simulink model "Copy_of_EMB_LRM_LaneRoleManager"  (R2025a)
settings: Solver=FixedStepDiscrete  StartTime=0.0  StopTime=inf  FixedStep=0.01  RelTol=1e-3
(part 1 of 2)
settings Model: Creator=wangtianqi  LastModifiedBy=wangtianqi

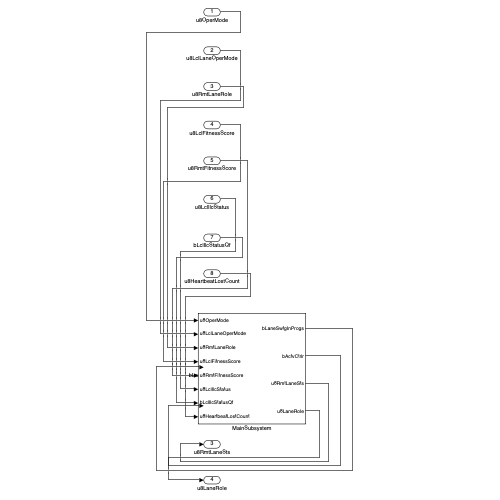
[thumbnail: Simulink's stored preview of the top-level diagram]
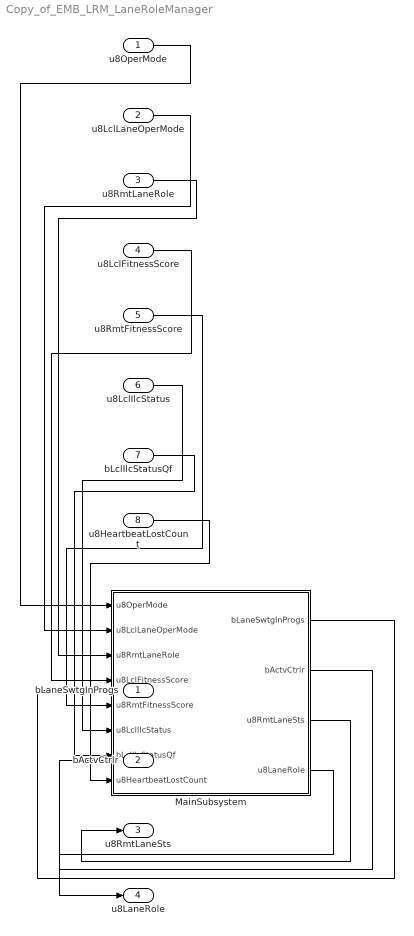
== system Copy_of_EMB_LRM_LaneRoleManager ==
  u8OperMode : Inport  Description=系统运行模式；类型 uint8；单位 -；范围 0..5 (0=OPMODE_INIT,1=OPMODE_NORMAL_OPERATION,2=OPMODE_LIMP_HOME,3=OPMODE_LIMP_ASIDE,4=OPMODE_CRAWL,5=OPMODE_SHUTTING_DOWN)  OutDataTypeStr=uint8
  u8LclLaneOperMode : Inport  Description=本控制链路运行模式；类型 uint8；单位 -；范围 0..5 (编码同系统运行模式)  Port=2  OutDataTypeStr=uint8
  u8RmtLaneRole : Inport  Description=远控制链路当前角色；类型 uint8；单位 -；范围 0..6 (0=UNKNOWN,1=INIT,2=MASTER,3=FALLBACK,4=SUPPORT,5=DISABLED,6=SHUTTING_DOWN)  Port=3  OutDataTypeStr=uint8
  u8LclFitnessScore : Inport  Description=本控制链路健康度得分；类型 uint8；单位 -；范围 0..255 (62=禁用,255=无效)  Port=4  OutDataTypeStr=uint8
  u8RmtFitnessScore : Inport  Description=远控制链路健康度得分；类型 uint8；单位 -；范围 0..255 (62=禁用,255=无效)  Port=5  OutDataTypeStr=uint8
  u8LclIlcStatus : Inport  Description=本控制链路 ILC 状态；类型 uint8；单位 -；范围 0..2 (0=Failed,1=Normal,2=Initialized)  Port=6  OutDataTypeStr=uint8
  bLclIlcStatusQf : Inport  Description=本控制链路 ILC 状态信号质量；类型 boolean；单位 -；范围 0..1 (1=QF_Not_Full 质量异常,0=QF_Full 质量正常)  Port=7  OutDataTypeStr=boolean
  u8HeartbeatLostCount : Inport  Description=心跳丢失计数；类型 uint8；单位 -；范围 0..255 (连续递增序列 0..255,0,1.. 表示正常)  Port=8  OutDataTypeStr=uint8
  MainSubsystem : Subsystem  Description=LRM 主包装子系统：信号采集 -> 链路状态管理(MLS) -> 角色仲裁(MLR) -> 切换防抖(LSP) -> 输出仲裁，实现 EMB 控制链路主从角色管理与切换标志输出
  bLaneSwtgInProgs : Outport  Description=控制链路切换进行中标志；类型 boolean；单位 -；范围 0..1 (0=Not Progress,1=Progress)
  bActvCtrlr : Outport  Description=活动控制器实例标志（本链路角色为 MASTER 时置 1）；类型 boolean；单位 -；范围 0..1 (0=Not Active,1=Active)  Port=2
  u8RmtLaneSts : Outport  Description=远控制链路状态（由远控角色与健康度映射派生）；类型 uint8；单位 -；范围 0..3 (0=INITIALISING,1=OPERATING,2=HB_LOST,3=FAILED)  Port=3
  u8LaneRole : Outport  Description=本控制链路角色状态；类型 uint8；单位 -；范围 0..6 (0=UNKNOWN,1=INIT,2=MASTER,3=FALLBACK,4=SUPPORT,5=DISABLED,6=SHUTTING_DOWN)  Port=4
  wires:
  u8OperMode/1 -> MainSubsystem/1(u8OperMode)
  u8LclLaneOperMode/1 -> MainSubsystem/2(u8LclLaneOperMode)
  u8RmtLaneRole/1 -> MainSubsystem/3(u8RmtLaneRole)
  u8LclFitnessScore/1 -> MainSubsystem/4(u8LclFitnessScore)
  u8RmtFitnessScore/1 -> MainSubsystem/5(u8RmtFitnessScore)
  u8LclIlcStatus/1 -> MainSubsystem/6(u8LclIlcStatus)
  bLclIlcStatusQf/1 -> MainSubsystem/7(bLclIlcStatusQf)
  u8HeartbeatLostCount/1 -> MainSubsystem/8(u8HeartbeatLostCount)
  MainSubsystem/1(bLaneSwtgInProgs) -> bLaneSwtgInProgs/1
  MainSubsystem/2(bActvCtrlr) -> bActvCtrlr/1
  MainSubsystem/3(u8RmtLaneSts) -> u8RmtLaneSts/1
  MainSubsystem/4(u8LaneRole) -> u8LaneRole/1

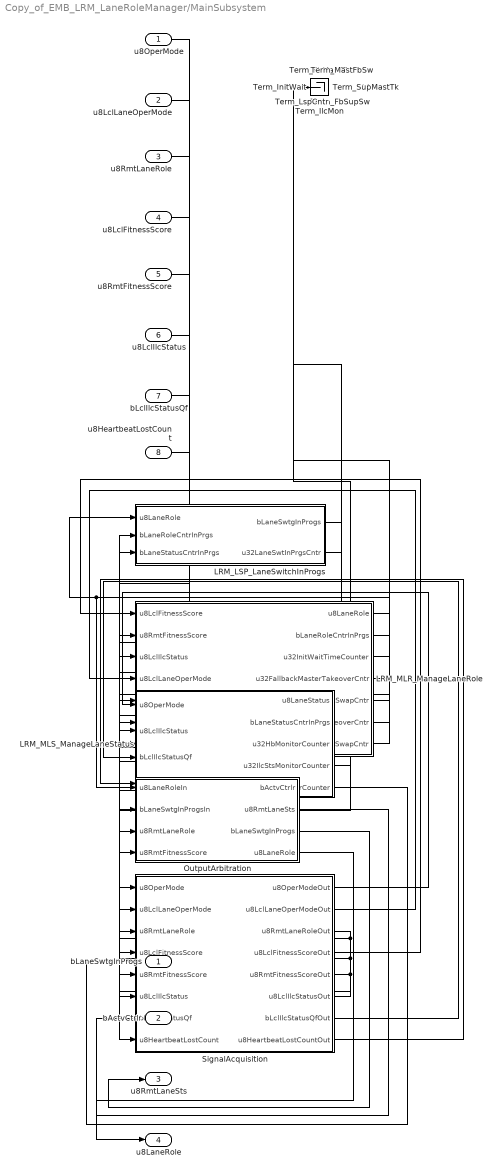
== system Copy_of_EMB_LRM_LaneRoleManager/MainSubsystem ==
  u8OperMode : Inport  Description=系统运行模式；类型 uint8；单位 -；范围 0..5  OutDataTypeStr=uint8
  u8LclLaneOperMode : Inport  Description=本控制链路运行模式；类型 uint8；单位 -；范围 0..5  Port=2  OutDataTypeStr=uint8
  u8RmtLaneRole : Inport  Description=远控制链路当前角色；类型 uint8；单位 -；范围 0..6  Port=3  OutDataTypeStr=uint8
  u8LclFitnessScore : Inport  Description=本控制链路健康度得分；类型 uint8；单位 -；范围 0..255 (62=禁用,255=无效)  Port=4  OutDataTypeStr=uint8
  u8RmtFitnessScore : Inport  Description=远控制链路健康度得分；类型 uint8；单位 -；范围 0..255 (62=禁用,255=无效)  Port=5  OutDataTypeStr=uint8
  u8LclIlcStatus : Inport  Description=本控制链路 ILC 状态；类型 uint8；单位 -；范围 0..2 (0=Failed,1=Normal,2=Initialized)  Port=6  OutDataTypeStr=uint8
  bLclIlcStatusQf : Inport  Description=本控制链路 ILC 状态信号质量；类型 boolean；单位 -；范围 0..1 (1=质量异常,0=质量正常)  Port=7  OutDataTypeStr=boolean
  u8HeartbeatLostCount : Inport  Description=心跳丢失计数；类型 uint8；单位 -；范围 0..255  Port=8  OutDataTypeStr=uint8
  LRM_LSP_LaneSwitchInProgs : Subsystem  Description=检测角色（LaneRole）变化并管理角色切换过渡过程（防抖），输出切换进行中标志与计数器；优先级 A>B>C：A=LaneRoleChanged 时 cntr=1,flag=1；B=cntr>0 时 cntr+1 并在超阈值后清零；C=IfAnyTimerNonZero 时 cntr=0,flag=1；由 Unit Delay / Sum / Switch 优先级链 / Relational Operator / Logical Operator 实现
  LRM_MLR_ManageLaneRole : Subsystem  Description=基于本/远控制链路健康度得分、ILC 状态、远控角色、LaneStatus 与运行模式仲裁本控制链路角色（INIT/DISABLED/SHUTTING_DOWN/SUPPORT/FALLBACK/MASTER）；内部含 MLR_STM（boolean-gated Stateflow，状态 Init/Disabled/ShuttingDown/OperationalRoles{Support,Fallback,Master}）与 Simulink 计数器（InitWaitTime/MasterFallbackSwap/FallbackMasterTakeover/FallbackSupportSwap/SupportMasterTakeover），条件全部在 Simulink 内计算为 boolean，图表仅输出 u8LaneRole
  LRM_MLS_ManageLaneStatus : Subsystem  Description=监控 LCL ILC STATUS_QF、OPER MODE 与 LCL ILC STATUS，结合心跳丢失判定输出控制链路健康状态 LaneStatus、状态切换标志与三个诊断计数器；内部含 MLS_HB_Failure（Unit Delay/Sum/Relational/Logic 组合）与 MLS_STM_StateMachine（boolean-gated Stateflow，状态 INIT.MonitoringOff/On、Operating、HbLost、Failed，优先级 Operating>Failed>HbLost；计数器与条件全部在 Simulink 内计算，图表仅接收 boolean 条件，输出 u8LaneStatus 与 bMonitoringActive）
  OutputArbitration : Subsystem  Description=输出仲裁与派生诊断：bActvCtrlr=(u8LaneRole==2)（Relational Operator）；u8RmtLaneSts 由 Switch 优先级链映射（DISABLED/SHUTTING_DOWN→FAILED、FITNESS==255→HB_LOST、UNKNOWN/INIT→INITIALISING、其余→OPERATING）；bLaneSwtgInProgs 与 u8LaneRole 直通
  SignalAcquisition : Subsystem  Description=信号调理与类型转换：全部顶层输入已采用内部一致表示（enum 用 uint8，质量标志用 boolean），无需类型转换，直通至下游；8 路输入与 8 路输出同名同类型一一对应，由同名 Inport/Outport 直连实现
  Term_FbMastTk : Terminator
      settings: Description=诊断计数器终止：u32FallbackMasterTakeoverCntr
  Term_FbSupSw : Terminator
      settings: Description=诊断计数器终止：u32FallbackSupportSwapCntr
  Term_HbMon : Terminator
      settings: Description=诊断计数器终止：u32HbMonitorCounter
  Term_IlcMon : Terminator
      settings: Description=诊断计数器终止：u32IlcStsMonitorCounter
  Term_InitWait : Terminator
      settings: Description=诊断计数器终止：u32InitWaitTimeCounter
  Term_LspCntr : Terminator
      settings: Description=诊断计数器终止：u32LaneSwtInPrgsCntr
  Term_MastFbSw : Terminator
      settings: Description=诊断计数器终止：u32MasterFallbackSwapCntr
  Term_SupMastTk : Terminator
      settings: Description=诊断计数器终止：u32SupportMasterTakeoverCntr
  bLaneSwtgInProgs : Outport  Description=控制链路切换进行中标志；类型 boolean；单位 -；范围 0..1
  bActvCtrlr : Outport  Description=活动控制器实例标志；类型 boolean；单位 -；范围 0..1  Port=2
  u8RmtLaneSts : Outport  Description=远控制链路状态；类型 uint8；单位 -；范围 0..3  Port=3
  u8LaneRole : Outport  Description=本控制链路角色状态；类型 uint8；单位 -；范围 0..6  Port=4
  wires:
  u8OperMode/1 -> SignalAcquisition/1(u8OperMode)
  u8LclLaneOperMode/1 -> SignalAcquisition/2(u8LclLaneOperMode)
  u8RmtLaneRole/1 -> SignalAcquisition/3(u8RmtLaneRole)
  u8LclFitnessScore/1 -> SignalAcquisition/4(u8LclFitnessScore)
  u8RmtFitnessScore/1 -> SignalAcquisition/5(u8RmtFitnessScore)
  u8LclIlcStatus/1 -> SignalAcquisition/6(u8LclIlcStatus)
  bLclIlcStatusQf/1 -> SignalAcquisition/7(bLclIlcStatusQf)
  u8HeartbeatLostCount/1 -> SignalAcquisition/8(u8HeartbeatLostCount)
  SignalAcquisition/1(u8OperModeOut) -> LRM_MLS_ManageLaneStatus/1(u8OperMode)
  SignalAcquisition/2(u8LclLaneOperModeOut) -> LRM_MLR_ManageLaneRole/4(u8LclLaneOperMode)
  SignalAcquisition/3(u8RmtLaneRoleOut) -> OutputArbitration/3(u8RmtLaneRole), LRM_MLR_ManageLaneRole/5(u8RmtLaneRole)
  SignalAcquisition/4(u8LclFitnessScoreOut) -> LRM_MLR_ManageLaneRole/1(u8LclFitnessScore)
  SignalAcquisition/5(u8RmtFitnessScoreOut) -> OutputArbitration/4(u8RmtFitnessScore), LRM_MLR_ManageLaneRole/2(u8RmtFitnessScore)
  SignalAcquisition/6(u8LclIlcStatusOut) -> LRM_MLR_ManageLaneRole/3(u8LclIlcStatus), LRM_MLS_ManageLaneStatus/2(u8LclIlcStatus)
  SignalAcquisition/7(bLclIlcStatusQfOut) -> LRM_MLS_ManageLaneStatus/3(bLclIlcStatusQf)
  SignalAcquisition/8(u8HeartbeatLostCountOut) -> LRM_MLS_ManageLaneStatus/4(u8HeartbeatLostCount)
  LRM_MLS_ManageLaneStatus/1(u8LaneStatus) -> LRM_MLR_ManageLaneRole/6(u8LaneStatus)
  LRM_MLS_ManageLaneStatus/2(bLaneStatusCntrInPrgs) -> LRM_LSP_LaneSwitchInProgs/3(bLaneStatusCntrInPrgs)
  LRM_MLS_ManageLaneStatus/3(u32HbMonitorCounter) -> Term_HbMon/1
  LRM_MLS_ManageLaneStatus/4(u32IlcStsMonitorCounter) -> Term_IlcMon/1
  LRM_MLS_ManageLaneStatus/5(u32FailureMonitorCounter) -> LRM_MLR_ManageLaneRole/7(u32FailureMonitorCounter)
  LRM_MLR_ManageLaneRole/1(u8LaneRole) -> LRM_LSP_LaneSwitchInProgs/1(u8LaneRole), OutputArbitration/1(u8LaneRoleIn)
  LRM_MLR_ManageLaneRole/2(bLaneRoleCntrInPrgs) -> LRM_LSP_LaneSwitchInProgs/2(bLaneRoleCntrInPrgs)
  LRM_MLR_ManageLaneRole/3(u32InitWaitTimeCounter) -> Term_InitWait/1
  LRM_MLR_ManageLaneRole/4(u32FallbackMasterTakeoverCntr) -> Term_FbMastTk/1
  LRM_MLR_ManageLaneRole/5(u32MasterFallbackSwapCntr) -> Term_MastFbSw/1
  LRM_MLR_ManageLaneRole/6(u32SupportMasterTakeoverCntr) -> Term_SupMastTk/1
  LRM_MLR_ManageLaneRole/7(u32FallbackSupportSwapCntr) -> Term_FbSupSw/1
  LRM_LSP_LaneSwitchInProgs/1(bLaneSwtgInProgs) -> OutputArbitration/2(bLaneSwtgInProgsIn)
  LRM_LSP_LaneSwitchInProgs/2(u32LaneSwtInPrgsCntr) -> Term_LspCntr/1
  OutputArbitration/1(bActvCtrlr) -> bLaneSwtgInProgs/1
  OutputArbitration/2(u8RmtLaneSts) -> bActvCtrlr/1
  OutputArbitration/3(bLaneSwtgInProgs) -> u8RmtLaneSts/1
  OutputArbitration/4(u8LaneRole) -> u8LaneRole/1

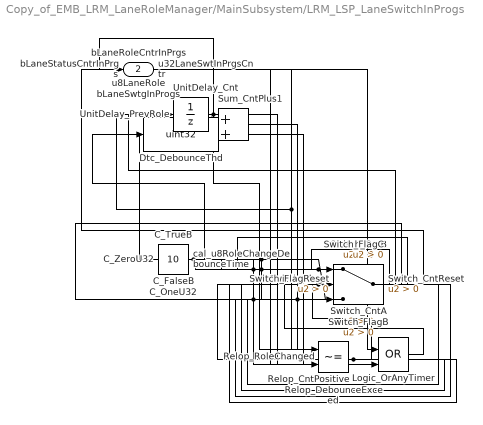
== system Copy_of_EMB_LRM_LaneRoleManager/MainSubsystem/LRM_LSP_LaneSwitchInProgs ==
  u8LaneRole : Inport  Description=当前周期角色决策值（来自 MLR）；类型 uint8；范围 0..6  OutDataTypeStr=uint8
  bLaneRoleCntrInPrgs : Inport  Description=角色切换计数器进行中标志（来自 MLR）；类型 boolean  Port=2  OutDataTypeStr=boolean
  bLaneStatusCntrInPrgs : Inport  Description=状态切换计数器进行中标志（来自 MLS）；类型 boolean  Port=3  OutDataTypeStr=boolean
  C_FalseB : Constant  Description=布尔假常量  Value=0  OutDataTypeStr=boolean
  C_OneU32 : Constant  Description=计数器步长 1；uint32  OutDataTypeStr=uint32
  C_TrueB : Constant  Description=布尔真常量  OutDataTypeStr=boolean
  C_ZeroU32 : Constant  Description=计数器清零常量；uint32  Value=0  OutDataTypeStr=uint32
  Dtc_DebounceThd : DataTypeConversion  Description=防抖阈值转 uint32  OutDataTypeStr=uint32  SaturateOnIntegerOverflow=off  RndMeth=Floor
  Logic_OrAnyTimer : Logic  Description=任一计时器进行中  Operator=OR  IconShape=distinctive  AllPortsSameDT=off  OutDataTypeStr=boolean
  Relop_CntPositive : RelationalOperator  Description=计数器 > 0（条件 B）  Operator=>  OutDataTypeStr=boolean  RndMeth=Simplest  InputSameDT=off
  Relop_DebounceExceed : RelationalOperator  Description=cnt+1 > 防抖阈值（清零条件）  Operator=>  OutDataTypeStr=boolean  RndMeth=Simplest  InputSameDT=off
  Relop_RoleChanged : RelationalOperator  Description=角色变化检测：当前角色 != 上一周期角色  Operator=~=  OutDataTypeStr=boolean  RndMeth=Simplest  InputSameDT=off
  Sum_CntPlus1 : Sum  Description=切换计数器 +1  Inputs=|++
  Switch_CntA : Switch  Description=A 优先级：角色变化置 1  Criteria=u2 > Threshold  SaturateOnIntegerOverflow=off  InputSameDT=off
  Switch_CntB : Switch  Description=B 分支门控：cnt>0 时按 B 处理，否则 0  Criteria=u2 > Threshold  SaturateOnIntegerOverflow=off  InputSameDT=off
  Switch_CntReset : Switch  Description=B 分支：超阈值清零，否则 +1  Criteria=u2 > Threshold  SaturateOnIntegerOverflow=off  InputSameDT=off
  Switch_FlagA : Switch  Description=标志 A 优先级：角色变化置 1  Criteria=u2 > Threshold  SaturateOnIntegerOverflow=off  InputSameDT=off
  Switch_FlagB : Switch  Description=标志 B 门控  Criteria=u2 > Threshold  SaturateOnIntegerOverflow=off  InputSameDT=off
  Switch_FlagC : Switch  Description=标志 C 分支：任一计时器进行中置 1  Criteria=u2 > Threshold  SaturateOnIntegerOverflow=off  InputSameDT=off
  Switch_FlagReset : Switch  Description=标志 B 分支：超阈值清零  Criteria=u2 > Threshold  SaturateOnIntegerOverflow=off  InputSameDT=off
  UnitDelay_Cnt : UnitDelay  Description=切换进行中计数器状态；uint32  SampleTime=-1  HasFrameUpgradeWarning=on
  UnitDelay_PrevRole : UnitDelay  Description=上一周期角色；uint8  SampleTime=-1  HasFrameUpgradeWarning=on
  cal_u8RoleChangeDebounceTime : Constant  Description=cal_u8RoleChangeDebounceTime；角色切换防抖时间阈值（周期数）；uint8；1..255；默认 10  Value=10  OutDataTypeStr=uint8
  bLaneSwtgInProgs : Outport  Description=控制链路切换进行中标志；类型 boolean；范围 0..1
  u32LaneSwtInPrgsCntr : Outport  Description=控制链路切换进行中计数器；类型 uint32  Port=2
  wires:
  u8LaneRole/1 -> UnitDelay_PrevRole/1, Relop_RoleChanged/1
  UnitDelay_PrevRole/1 -> Relop_RoleChanged/2
  bLaneRoleCntrInPrgs/1 -> Logic_OrAnyTimer/1
  bLaneStatusCntrInPrgs/1 -> Logic_OrAnyTimer/2
  UnitDelay_Cnt/1 -> Relop_CntPositive/1, Sum_CntPlus1/1, u32LaneSwtInPrgsCntr/1
  C_OneU32/1 -> Switch_CntA/1, Sum_CntPlus1/2
  C_ZeroU32/1 -> Switch_CntB/3, Relop_CntPositive/2, Switch_CntReset/1
  cal_u8RoleChangeDebounceTime/1 -> Dtc_DebounceThd/1
  Dtc_DebounceThd/1 -> Relop_DebounceExceed/2
  Sum_CntPlus1/1 -> Switch_CntReset/3, Relop_DebounceExceed/1
  Relop_DebounceExceed/1 -> Switch_FlagReset/2, Switch_CntReset/2
  Switch_CntReset/1 -> Switch_CntB/1
  Relop_CntPositive/1 -> Switch_FlagB/2, Switch_CntB/2
  Relop_RoleChanged/1 -> Switch_FlagA/2, Switch_CntA/2
  Switch_CntB/1 -> Switch_CntA/3
  Switch_CntA/1 -> UnitDelay_Cnt/1
  C_FalseB/1 -> Switch_FlagC/3, Switch_FlagReset/1
  C_TrueB/1 -> Switch_FlagA/1, Switch_FlagC/1, Switch_FlagReset/3
  Switch_FlagReset/1 -> Switch_FlagB/1
  Switch_FlagC/1 -> Switch_FlagB/3
  Logic_OrAnyTimer/1 -> Switch_FlagC/2
  Switch_FlagB/1 -> Switch_FlagA/3
  Switch_FlagA/1 -> bLaneSwtgInProgs/1

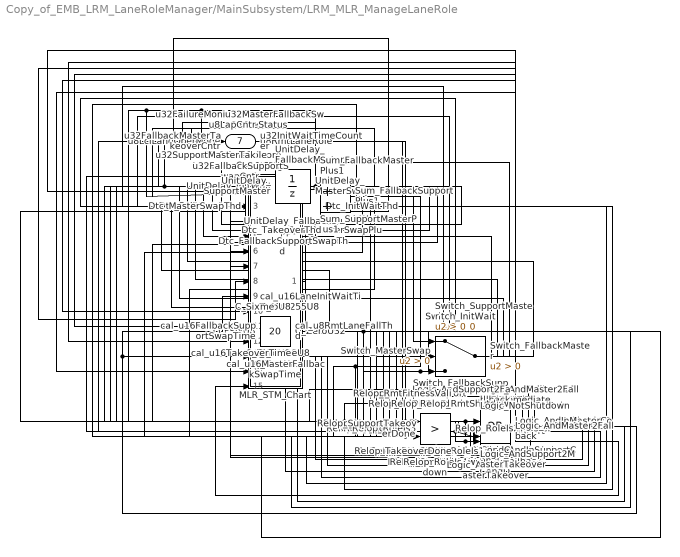
== system Copy_of_EMB_LRM_LaneRoleManager/MainSubsystem/LRM_MLR_ManageLaneRole ==
  u8LclFitnessScore : Inport  Description=本控制链路健康度得分；类型 uint8；范围 0..255 (62=禁用,255=无效)  OutDataTypeStr=uint8
  u8RmtFitnessScore : Inport  Description=远控制链路健康度得分；类型 uint8；范围 0..255 (62=禁用,255=无效)  Port=2  OutDataTypeStr=uint8
  u8LclIlcStatus : Inport  Description=本控制链路 ILC 状态；类型 uint8；范围 0..2 (0=Failed,1=Normal,2=Initialized)  Port=3  OutDataTypeStr=uint8
  u8LclLaneOperMode : Inport  Description=本控制链路运行模式；类型 uint8；范围 0..5  Port=4  OutDataTypeStr=uint8
  u8RmtLaneRole : Inport  Description=远控制链路当前角色；类型 uint8；范围 0..6  Port=5  OutDataTypeStr=uint8
  u8LaneStatus : Inport  Description=控制链路健康状态（来自 MLS）；类型 uint8；范围 0..3  Port=6  OutDataTypeStr=uint8
  u32FailureMonitorCounter : Inport  Description=故障监控计数器（来自 MLS）；类型 uint32  Port=7  OutDataTypeStr=uint32
  C_FiveU8 : Constant  Description=常量 5（LN_ROLE_DISABLED）；uint8  Value=5  OutDataTypeStr=uint8
  C_FourU8 : Constant  Description=常量 4（LN_ROLE_SUPPORT）；uint8  Value=4  OutDataTypeStr=uint8
  C_Max255U8 : Constant  Description=健康度无效值 255；uint8  Value=255  OutDataTypeStr=uint8
  C_OneU32 : Constant  Description=计数器步长 1；uint32  OutDataTypeStr=uint32
  C_OneU8 : Constant  Description=常量 1（LN_ROLE_INIT）；uint8  OutDataTypeStr=uint8
  C_SixTwoU8 : Constant  Description=健康度禁用值 62；uint8  Value=62  OutDataTypeStr=uint8
  C_SixU8 : Constant  Description=常量 6（LN_ROLE_SHUTTING_DOWN）；uint8  Value=6  OutDataTypeStr=uint8
  C_ThreeU8 : Constant  Description=常量 3（LN_ROLE_FALLBACK）；uint8  Value=3  OutDataTypeStr=uint8
  C_TwoU8 : Constant  Description=常量 2（LN_ROLE_MASTER）；uint8  Value=2  OutDataTypeStr=uint8
  C_ZeroU32 : Constant  Description=计数器清零常量；uint32  Value=0  OutDataTypeStr=uint32
  C_ZeroU8 : Constant  Description=零常量；uint8  Value=0  OutDataTypeStr=uint8
  Dtc_FailWatchThd : DataTypeConversion  Description=故障监控阈值转 uint32  OutDataTypeStr=uint32  SaturateOnIntegerOverflow=off  RndMeth=Floor
  Dtc_FallbackSupportSwapThd : DataTypeConversion  Description=FallbackSupportSwap 阈值转 uint32  OutDataTypeStr=uint32  SaturateOnIntegerOverflow=off  RndMeth=Floor
  Dtc_InitWaitThd : DataTypeConversion  Description=InitWait 阈值转 uint32  OutDataTypeStr=uint32  SaturateOnIntegerOverflow=off  RndMeth=Floor
  Dtc_MasterSwapThd : DataTypeConversion  Description=MasterSwap 阈值转 uint32  OutDataTypeStr=uint32  SaturateOnIntegerOverflow=off  RndMeth=Floor
  Dtc_TakeoverThd : DataTypeConversion  Description=接管阈值转 uint32  OutDataTypeStr=uint32  SaturateOnIntegerOverflow=off  RndMeth=Floor
  Logic_AndArbLcl : Logic  Description=仲裁条件（本地更优）：等待完成 且 本地>远程  IconShape=distinctive  AllPortsSameDT=off  OutDataTypeStr=boolean
  Logic_AndCondA : Logic  Description=条件A：ILC 故障 且 远程有效 且 本地<远程（Master->Support 直接降级）  Inputs=3  IconShape=distinctive  AllPortsSameDT=off  OutDataTypeStr=boolean
  Logic_AndCondD : Logic  Description=条件D：本地>远程 且 远程有效（接管条件，假设）  IconShape=distinctive  AllPortsSameDT=off  OutDataTypeStr=boolean
  Logic_AndFallback2MasterTakeover : Logic  Description=Fallback->Master（接管）：条件D 且 计数超阈值 且 远程非MASTER  Inputs=3  IconShape=distinctive  AllPortsSameDT=off  OutDataTypeStr=boolean
  Logic_AndFallback2Support : Logic  Description=Fallback->Support：条件E 且 计数超阈值  IconShape=distinctive  AllPortsSameDT=off  OutDataTypeStr=boolean
  Logic_AndFallback2SupportUnknown : Logic  Description=Fallback->Support：远程UNKNOWN 且 故障监控超窗  IconShape=distinctive  AllPortsSameDT=off  OutDataTypeStr=boolean
  Logic_AndInFallbackCondD : Logic  Description=Fallback 内条件D持续  IconShape=distinctive  AllPortsSameDT=off  OutDataTypeStr=boolean
  Logic_AndInFallbackCondE : Logic  Description=Fallback 内条件E持续  IconShape=distinctive  AllPortsSameDT=off  OutDataTypeStr=boolean
  Logic_AndInMasterCondB : Logic  Description=Master 内条件B持续  IconShape=distinctive  AllPortsSameDT=off  OutDataTypeStr=boolean
  Logic_AndInSupportCondG : Logic  Description=Support 内条件G持续  IconShape=distinctive  AllPortsSameDT=off  OutDataTypeStr=boolean
  Logic_AndMaster2Fallback : Logic  Description=Master->Fallback：条件B持续 且 远程FALLBACK 且 计数超阈值  Inputs=3  IconShape=distinctive  AllPortsSameDT=off  OutDataTypeStr=boolean
  Logic_AndMaster2FallbackImmediate : Logic  Description=Master->Fallback（立即）：条件B 且 远程MASTER  IconShape=distinctive  AllPortsSameDT=off  OutDataTypeStr=boolean
  Logic_AndSupport2Fallback : Logic  Description=Support->Fallback（恢复）：ILC 非故障 且 远程MASTER  IconShape=distinctive  AllPortsSameDT=off  OutDataTypeStr=boolean
  Logic_AndSupport2MasterTakeover : Logic  Description=Support->Master（接管）：条件G 且 计数超阈值 且 远程非MASTER  Inputs=3  IconShape=distinctive  AllPortsSameDT=off  OutDataTypeStr=boolean
  Logic_NotIlcFailed : Logic  Description=ILC 非 Failed  Operator=NOT  Inputs=1  IconShape=distinctive  AllPortsSameDT=off  OutDataTypeStr=boolean
  Logic_NotShutdown : Logic  Description=非关闭模式  Operator=NOT  Inputs=1  IconShape=distinctive  AllPortsSameDT=off  OutDataTypeStr=boolean
  Logic_OrCondC : Logic  Description=条件C：LaneStatus==FAILED 或 远程禁用/关闭  Operator=OR  IconShape=distinctive  AllPortsSameDT=off  OutDataTypeStr=boolean
  Logic_OrRmtDisShut : Logic  Description=远程禁用或关闭  Operator=OR  IconShape=distinctive  AllPortsSameDT=off  OutDataTypeStr=boolean
  MLR_STM_Chart : Stateflow chart  Description=MLR_STM 布尔门控 Stateflow：输入全为 boolean 条件（15 路），输出 u8LaneRole；状态 Init/Disabled/ShuttingDown/OperationalRoles{Support,FallBack,Master}  TreatAsAtomicUnit=on
  Relop_FailWatchDone : RelationalOperator  Description=FailureMonitorCounter > 窗口阈值  Operator=>  OutDataTypeStr=boolean  RndMeth=Simplest  InputSameDT=off
  Relop_FallbackSwapDone : RelationalOperator  Description=FallbackSupportSwapCntr > 阈值  Operator=>  OutDataTypeStr=boolean  RndMeth=Simplest  InputSameDT=off
  Relop_IlcFailed : RelationalOperator  Description=ILC 状态==Failed  Operator===  OutDataTypeStr=boolean  RndMeth=Simplest  InputSameDT=off
  Relop_InitWaitDone : RelationalOperator  Description=InitWaitTime >= 阈值  Operator=<=  OutDataTypeStr=boolean  RndMeth=Simplest  InputSameDT=off
  Relop_LaneOperShutdown : RelationalOperator  Description=本链路运行模式==SHUTTING_DOWN  Operator===  OutDataTypeStr=boolean  RndMeth=Simplest  InputSameDT=off
  Relop_LaneStsFailed : RelationalOperator  Description=LaneStatus==FAILED  Operator===  OutDataTypeStr=boolean  RndMeth=Simplest  InputSameDT=off
  Relop_LclDisabled : RelationalOperator  Description=本链路健康度==62（禁用）  Operator===  OutDataTypeStr=boolean  RndMeth=Simplest  InputSameDT=off
  Relop_LclGtRmt : RelationalOperator  Description=本链路健康度 > 远程  Operator=>  OutDataTypeStr=boolean  RndMeth=Simplest  InputSameDT=off
  Relop_LclLtRmt : RelationalOperator  Description=本链路健康度 < 远程  Operator=<  OutDataTypeStr=boolean  RndMeth=Simplest  InputSameDT=off
  Relop_MasterSwapDone : RelationalOperator  Description=MasterSwapCntr > 阈值  Operator=>  OutDataTypeStr=boolean  RndMeth=Simplest  InputSameDT=off
  Relop_RmtDisabled : RelationalOperator  Description=远程角色==DISABLED  Operator===  OutDataTypeStr=boolean  RndMeth=Simplest  InputSameDT=off
  Relop_RmtFallback : RelationalOperator  Description=远程角色==FALLBACK  Operator===  OutDataTypeStr=boolean  RndMeth=Simplest  InputSameDT=off
  Relop_RmtFitnessValid : RelationalOperator  Description=远程健康度非无效(255)  Operator=~=  OutDataTypeStr=boolean  RndMeth=Simplest  InputSameDT=off
  Relop_RmtMaster : RelationalOperator  Description=远程角色==MASTER  Operator===  OutDataTypeStr=boolean  RndMeth=Simplest  InputSameDT=off
  Relop_RmtNotMaster : RelationalOperator  Description=远程角色非 MASTER  Operator=~=  OutDataTypeStr=boolean  RndMeth=Simplest  InputSameDT=off
  Relop_RmtShutdown : RelationalOperator  Description=远程角色==SHUTTING_DOWN  Operator===  OutDataTypeStr=boolean  RndMeth=Simplest  InputSameDT=off
  Relop_RmtUnknown : RelationalOperator  Description=远程角色==UNKNOWN  Operator===  OutDataTypeStr=boolean  RndMeth=Simplest  InputSameDT=off
  Relop_RoleIs1 : RelationalOperator  Description=当前角色==INIT  Operator===  OutDataTypeStr=boolean  RndMeth=Simplest  InputSameDT=off
  Relop_RoleIs2 : RelationalOperator  Description=当前角色==MASTER  Operator===  OutDataTypeStr=boolean  RndMeth=Simplest  InputSameDT=off
  Relop_RoleIs3 : RelationalOperator  Description=当前角色==FALLBACK  Operator===  OutDataTypeStr=boolean  RndMeth=Simplest  InputSameDT=off
  Relop_RoleIs4 : RelationalOperator  Description=当前角色==SUPPORT  Operator===  OutDataTypeStr=boolean  RndMeth=Simplest  InputSameDT=off
  Relop_SupportTakeoverDone : RelationalOperator  Description=SupportMasterTakeoverCntr > 阈值  Operator=>  OutDataTypeStr=boolean  RndMeth=Simplest  InputSameDT=off
  Relop_TakeoverDone : RelationalOperator  Description=FallbackMasterTakeoverCntr > 阈值  Operator=>  OutDataTypeStr=boolean  RndMeth=Simplest  InputSameDT=off
  Sum_FallbackMasterPlus1 : Sum  Description=FallbackMaster 计数器 +1  Inputs=|++
  Sum_FallbackSupportPlus1 : Sum  Description=FallbackSupport 计数器 +1  Inputs=|++
  Sum_InitWaitPlus1 : Sum  Description=InitWait 计数器 +1  Inputs=|++
  Sum_MasterSwapPlus1 : Sum  Description=MasterSwap 计数器 +1  Inputs=|++
  Sum_SupportMasterPlus1 : Sum  Description=SupportMaster 计数器 +1  Inputs=|++
  Switch_FallbackMaster : Switch  Description=Fallback 内条件D持续时计数，否则清零  Criteria=u2 > Threshold  SaturateOnIntegerOverflow=off  InputSameDT=off
  Switch_FallbackSupport : Switch  Description=Fallback 内条件E持续时计数，否则清零  Criteria=u2 > Threshold  SaturateOnIntegerOverflow=off  InputSameDT=off
  Switch_InitWait : Switch  Description=Init 状态内计数，否则清零  Criteria=u2 > Threshold  SaturateOnIntegerOverflow=off  InputSameDT=off
  Switch_MasterSwap : Switch  Description=Master 内条件B持续时计数，否则清零  Criteria=u2 > Threshold  SaturateOnIntegerOverflow=off  InputSameDT=off
  Switch_SupportMaster : Switch  Description=Support 内条件G持续时计数，否则清零  Criteria=u2 > Threshold  SaturateOnIntegerOverflow=off  InputSameDT=off
  UnitDelay_FallbackMaster : UnitDelay  Description=Fallback->Master 接管计数器；uint32  SampleTime=-1  HasFrameUpgradeWarning=on
  UnitDelay_FallbackSupport : UnitDelay  Description=Fallback->Support 切换计数器；uint32  SampleTime=-1  HasFrameUpgradeWarning=on
  UnitDelay_InitWait : UnitDelay  Description=初始化等待计数器状态；uint32  SampleTime=-1  HasFrameUpgradeWarning=on
  UnitDelay_MasterSwap : UnitDelay  Description=Master->Fallback 切换计数器；uint32  SampleTime=-1  HasFrameUpgradeWarning=on
  UnitDelay_SupportMaster : UnitDelay  Description=Support->Master 接管计数器；uint32  SampleTime=-1  HasFrameUpgradeWarning=on
  cal_u16FallbackSupportSwapTime : Constant  Description=cal_u16FallbackSupportSwapTime；Fallback->Support 切换阈值；uint16；1..65535；默认 20（假设值）  Value=20  OutDataTypeStr=uint16
  cal_u16LaneInitWaitTime : Constant  Description=cal_u16LaneInitWaitTime；初始化等待时间阈值（周期数）；uint16；1..65535；默认 100（假设值，文档未给初值）  Value=100  OutDataTypeStr=uint16
  cal_u16MasterFallbackSwapTime : Constant  Description=cal_u16MasterFallbackSwapTime；Master->Fallback 切换阈值；uint16；1..65535；默认 20  Value=20  OutDataTypeStr=uint16
  cal_u16TakeoverTime : Constant  Description=cal_u16TakeoverTime；接管计数阈值（周期数）；uint16；1..65535；默认 50（假设值）  Value=50  OutDataTypeStr=uint16
  cal_u8RmtLaneFallThd : Constant  Description=cal_u8RmtLaneFallThd；故障监控窗口阈值（周期数）；uint8；1..255；默认 20  Value=20  OutDataTypeStr=uint8
  u8LaneRole : Outport  Description=本控制链路角色决策结果；类型 uint8；范围 0..6
  bLaneRoleCntrInPrgs : Outport  Description=角色切换计数器进行中标志；类型 boolean  Port=2
  u32InitWaitTimeCounter : Outport  Description=初始化等待计数器；类型 uint32  Port=3
  u32FallbackMasterTakeoverCntr : Outport  Description=Fallback->Master 接管计数器；类型 uint32  Port=4
  u32MasterFallbackSwapCntr : Outport  Description=Master->Fallback 切换计数器；类型 uint32  Port=5
  u32SupportMasterTakeoverCntr : Outport  Description=Support->Master 接管计数器；类型 uint32  Port=6
  u32FallbackSupportSwapCntr : Outport  Description=Fallback->Support 切换计数器；类型 uint32  Port=7
  wires:
  u8LclFitnessScore/1 -> Relop_LclLtRmt/1, Relop_LclGtRmt/1, Relop_LclDisabled/1
  u8RmtFitnessScore/1 -> Relop_LclLtRmt/2, Relop_LclGtRmt/2, Relop_RmtFitnessValid/1
  u8LclIlcStatus/1 -> Relop_IlcFailed/1
  u8LclLaneOperMode/1 -> Relop_LaneOperShutdown/1
  u8RmtLaneRole/1 -> Relop_RmtUnknown/1, Relop_RmtShutdown/1, Relop_RmtDisabled/1, Relop_RmtNotMaster/1, Relop_RmtFallback/1, Relop_RmtMaster/1
  u8LaneStatus/1 -> Relop_LaneStsFailed/1
  u32FailureMonitorCounter/1 -> Relop_FailWatchDone/1
  C_SixTwoU8/1 -> Relop_LclDisabled/2
  C_Max255U8/1 -> Relop_RmtFitnessValid/2
  C_ZeroU8/1 -> Relop_RmtUnknown/2, Relop_IlcFailed/2
  C_FiveU8/1 -> Relop_RmtDisabled/2, Relop_LaneOperShutdown/2
  C_SixU8/1 -> Relop_RmtShutdown/2
  C_TwoU8/1 -> Relop_RoleIs2/2, Relop_RmtNotMaster/2, Relop_RmtMaster/2
  C_ThreeU8/1 -> Relop_RoleIs3/2, Relop_LaneStsFailed/2, Relop_RmtFallback/2
  Relop_LaneOperShutdown/1 -> Logic_NotShutdown/1, MLR_STM_Chart/1(bShutdown)
  Relop_RmtDisabled/1 -> Logic_OrRmtDisShut/1
  Relop_RmtShutdown/1 -> Logic_OrRmtDisShut/2
  Relop_LaneStsFailed/1 -> Logic_OrCondC/1
  Logic_OrRmtDisShut/1 -> Logic_OrCondC/2
  Relop_IlcFailed/1 -> Logic_AndInFallbackCondE/2, Logic_AndFallback2Support/1, Logic_AndCondA/1, Logic_NotIlcFailed/1
  Relop_RmtFitnessValid/1 -> Logic_AndCondD/2, Logic_AndCondA/2
  Relop_LclLtRmt/1 -> Logic_AndInMasterCondB/2, Logic_AndMaster2FallbackImmediate/1, Logic_AndMaster2Fallback/1, Logic_AndCondA/3
  Relop_LclGtRmt/1 -> Logic_AndArbLcl/2, Logic_AndCondD/1
  Relop_RmtFallback/1 -> Logic_AndMaster2Fallback/2
  Relop_MasterSwapDone/1 -> Logic_AndMaster2Fallback/3
  Relop_RmtMaster/1 -> Logic_AndSupport2Fallback/2, Logic_AndMaster2FallbackImmediate/2, MLR_STM_Chart/5(bArbRmtMaster)
  Logic_AndCondD/1 -> Logic_AndInSupportCondG/2, Logic_AndInFallbackCondD/2, Logic_AndSupport2MasterTakeover/1, Logic_AndFallback2MasterTakeover/1
  Relop_TakeoverDone/1 -> Logic_AndFallback2MasterTakeover/2
  Relop_RmtNotMaster/1 -> Logic_AndSupport2MasterTakeover/3, Logic_AndFallback2MasterTakeover/3
  Relop_FallbackSwapDone/1 -> Logic_AndFallback2Support/2
  Relop_RmtUnknown/1 -> Logic_AndFallback2SupportUnknown/1
  Relop_FailWatchDone/1 -> Logic_AndFallback2SupportUnknown/2
  Relop_SupportTakeoverDone/1 -> Logic_AndSupport2MasterTakeover/2
  Logic_NotIlcFailed/1 -> Logic_AndSupport2Fallback/1
  UnitDelay_InitWait/1 -> Relop_InitWaitDone/1, Sum_InitWaitPlus1/1, u32InitWaitTimeCounter/1
  C_OneU32/1 -> Sum_SupportMasterPlus1/2, Sum_FallbackSupportPlus1/2, Sum_FallbackMasterPlus1/2, Sum_MasterSwapPlus1/2, Sum_InitWaitPlus1/2
  Sum_InitWaitPlus1/1 -> Switch_InitWait/1
  Relop_RoleIs1/1 -> bLaneRoleCntrInPrgs/1, Switch_InitWait/2
  C_ZeroU32/1 -> Switch_SupportMaster/3, Switch_FallbackSupport/3, Switch_FallbackMaster/3, Switch_MasterSwap/3, Switch_InitWait/3
  Switch_InitWait/1 -> UnitDelay_InitWait/1
  Relop_RoleIs2/1 -> Logic_AndInMasterCondB/1
  UnitDelay_MasterSwap/1 -> Relop_MasterSwapDone/1, u32MasterFallbackSwapCntr/1, Sum_MasterSwapPlus1/1
  Sum_MasterSwapPlus1/1 -> Switch_MasterSwap/1
  Logic_AndInMasterCondB/1 -> Switch_MasterSwap/2
  Switch_MasterSwap/1 -> UnitDelay_MasterSwap/1
  Relop_RoleIs3/1 -> Logic_AndInFallbackCondE/1, Logic_AndInFallbackCondD/1
  UnitDelay_FallbackMaster/1 -> Relop_TakeoverDone/1, u32FallbackMasterTakeoverCntr/1, Sum_FallbackMasterPlus1/1
  Sum_FallbackMasterPlus1/1 -> Switch_FallbackMaster/1
  Logic_AndInFallbackCondD/1 -> Switch_FallbackMaster/2
  Switch_FallbackMaster/1 -> UnitDelay_FallbackMaster/1
  UnitDelay_FallbackSupport/1 -> Relop_FallbackSwapDone/1, u32FallbackSupportSwapCntr/1, Sum_FallbackSupportPlus1/1
  Sum_FallbackSupportPlus1/1 -> Switch_FallbackSupport/1
  Logic_AndInFallbackCondE/1 -> Switch_FallbackSupport/2
  Switch_FallbackSupport/1 -> UnitDelay_FallbackSupport/1
  Relop_RoleIs4/1 -> Logic_AndInSupportCondG/1
  UnitDelay_SupportMaster/1 -> Relop_SupportTakeoverDone/1, u32SupportMasterTakeoverCntr/1, Sum_SupportMasterPlus1/1
  Sum_SupportMasterPlus1/1 -> Switch_SupportMaster/1
  Logic_AndInSupportCondG/1 -> Switch_SupportMaster/2
  Switch_SupportMaster/1 -> UnitDelay_SupportMaster/1
  cal_u16LaneInitWaitTime/1 -> Dtc_InitWaitThd/1
  Dtc_InitWaitThd/1 -> Relop_InitWaitDone/2
  Relop_InitWaitDone/1 -> Logic_AndArbLcl/1
  cal_u16MasterFallbackSwapTime/1 -> Dtc_MasterSwapThd/1
  Dtc_MasterSwapThd/1 -> Relop_MasterSwapDone/2
  cal_u16TakeoverTime/1 -> Dtc_TakeoverThd/1
  Dtc_TakeoverThd/1 -> Relop_SupportTakeoverDone/2, Relop_TakeoverDone/2
  cal_u16FallbackSupportSwapTime/1 -> Dtc_FallbackSupportSwapThd/1
  Dtc_FallbackSupportSwapThd/1 -> Relop_FallbackSwapDone/2
  cal_u8RmtLaneFallThd/1 -> Dtc_FailWatchThd/1
  Dtc_FailWatchThd/1 -> Relop_FailWatchDone/2
  Logic_NotShutdown/1 -> MLR_STM_Chart/2(bNotShutdown)
  Relop_LclDisabled/1 -> MLR_STM_Chart/3(bLclDisabled)
  Logic_AndArbLcl/1 -> MLR_STM_Chart/4(bArbLclGtRmt)
  Logic_AndCondA/1 -> MLR_STM_Chart/6(bMaster2Support)
  Logic_AndMaster2Fallback/1 -> MLR_STM_Chart/7(bMaster2Fallback)
  Logic_AndMaster2FallbackImmediate/1 -> MLR_STM_Chart/8(bMaster2FallbackImmediate)
  Logic_OrCondC/1 -> MLR_STM_Chart/9(bFallback2Master), MLR_STM_Chart/13(bSupport2Master)
  Logic_AndFallback2MasterTakeover/1 -> MLR_STM_Chart/10(bFallback2MasterTakeover)
  Logic_AndFallback2Support/1 -> MLR_STM_Chart/11(bFallback2Support)
  Logic_AndFallback2SupportUnknown/1 -> MLR_STM_Chart/12(bFallback2SupportUnknown)
  Logic_AndSupport2MasterTakeover/1 -> MLR_STM_Chart/14(bSupport2MasterTakeover)
  Logic_AndSupport2Fallback/1 -> MLR_STM_Chart/15(bSupport2Fallback)
  MLR_STM_Chart/1(u8LaneRole) -> Relop_RoleIs4/1, Relop_RoleIs3/1, Relop_RoleIs2/1, Relop_RoleIs1/1, u8LaneRole/1
  C_OneU8/1 -> Relop_RoleIs1/2
  C_FourU8/1 -> Relop_RoleIs4/2

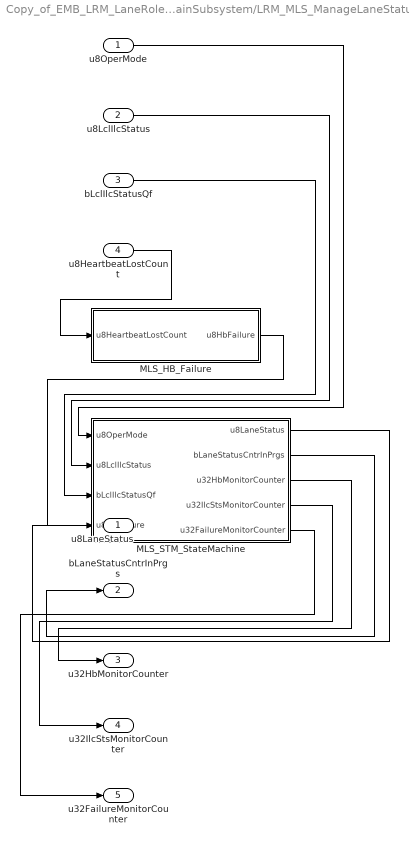
== system Copy_of_EMB_LRM_LaneRoleManager/MainSubsystem/LRM_MLS_ManageLaneStatus ==
  u8OperMode : Inport  Description=系统运行模式；类型 uint8；范围 0..5  OutDataTypeStr=uint8
  u8LclIlcStatus : Inport  Description=本控制链路 ILC 状态；类型 uint8；范围 0..2 (0=Failed,1=Normal,2=Initialized)  Port=2  OutDataTypeStr=uint8
  bLclIlcStatusQf : Inport  Description=本控制链路 ILC 状态信号质量；类型 boolean；范围 0..1 (1=异常,0=正常)  Port=3  OutDataTypeStr=boolean
  u8HeartbeatLostCount : Inport  Description=心跳丢失计数；类型 uint8；范围 0..255  Port=4  OutDataTypeStr=uint8
  MLS_HB_Failure : Subsystem  Description=MLS_HB_Failure 心跳丢失判定：HEARTBEAT LOST COUNT 连续递增(0..255,0,1..) 时 u8HbFailure=0，否则=1；由 Unit Delay 保存上一周期值，Sum/Relational Operator/Logical Operator 组合实现
  MLS_STM_StateMachine : Subsystem  Description=MLS_STM_StateMachine LaneStatus 状态机：条件与计数器全部在 Simulink 内计算（bMonitoringActive/bHlthOk/bHbLostCond/bFailedCond、Hb/ILC/Failure 三个 u32 计数器），boolean-gated Stateflow 实现 INIT.MonitoringOff/On、Operating、HbLost、Failed 状态转移（优先级 Operating>Failed>HbLost），图表输出 u8LaneStatus 与 bMonActive
  u8LaneStatus : Outport  Description=控制链路健康状态；类型 uint8；范围 0..3 (0=INITIALISING,1=OPERATING,2=HB_LOST,3=FAILED)
  bLaneStatusCntrInPrgs : Outport  Description=状态切换计数器进行中标志；类型 boolean；范围 0..1  Port=2
  u32HbMonitorCounter : Outport  Description=心跳监控计数器（诊断）；类型 uint32  Port=3
  u32IlcStsMonitorCounter : Outport  Description=ILC 状态监控计数器（诊断）；类型 uint32  Port=4
  u32FailureMonitorCounter : Outport  Description=故障监控计数器（诊断/供 MLR 使用）；类型 uint32  Port=5
  wires:
  u8OperMode/1 -> MLS_STM_StateMachine/1(u8OperMode)
  u8LclIlcStatus/1 -> MLS_STM_StateMachine/2(u8LclIlcStatus)
  bLclIlcStatusQf/1 -> MLS_STM_StateMachine/3(bLclIlcStatusQf)
  u8HeartbeatLostCount/1 -> MLS_HB_Failure/1(u8HeartbeatLostCount)
  MLS_HB_Failure/1(u8HbFailure) -> MLS_STM_StateMachine/4(u8HbFailure)
  MLS_STM_StateMachine/1(u8LaneStatus) -> u8LaneStatus/1
  MLS_STM_StateMachine/2(bLaneStatusCntrInPrgs) -> bLaneStatusCntrInPrgs/1
  MLS_STM_StateMachine/3(u32HbMonitorCounter) -> u32HbMonitorCounter/1
  MLS_STM_StateMachine/4(u32IlcStsMonitorCounter) -> u32IlcStsMonitorCounter/1
  MLS_STM_StateMachine/5(u32FailureMonitorCounter) -> u32FailureMonitorCounter/1

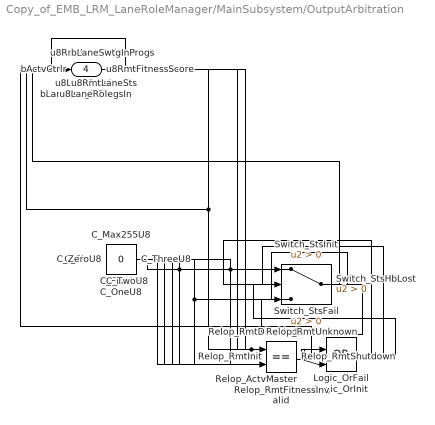
== system Copy_of_EMB_LRM_LaneRoleManager/MainSubsystem/OutputArbitration ==
  u8LaneRoleIn : Inport  Description=本控制链路角色（来自 MLR）；类型 uint8；范围 0..6  OutDataTypeStr=uint8
  bLaneSwtgInProgsIn : Inport  Description=控制链路切换进行中标志（来自 LSP）；类型 boolean  Port=2  OutDataTypeStr=boolean
  u8RmtLaneRole : Inport  Description=远控制链路当前角色；类型 uint8；范围 0..6  Port=3  OutDataTypeStr=uint8
  u8RmtFitnessScore : Inport  Description=远控制链路健康度得分；类型 uint8；范围 0..255  Port=4  OutDataTypeStr=uint8
  C_FiveU8 : Constant  Description=常量 5（LN_ROLE_DISABLED）；uint8  Value=5  OutDataTypeStr=uint8
  C_Max255U8 : Constant  Description=常量 255（健康度无效）；uint8  Value=255  OutDataTypeStr=uint8
  C_OneU8 : Constant  Description=常量 1（LANE_STS_OPERATING）；uint8  OutDataTypeStr=uint8
  C_SixU8 : Constant  Description=常量 6（LN_ROLE_SHUTTING_DOWN）；uint8  Value=6  OutDataTypeStr=uint8
  C_ThreeU8 : Constant  Description=常量 3（LANE_STS_FAILED）；uint8  Value=3  OutDataTypeStr=uint8
  C_TwoU8 : Constant  Description=常量 2（LN_ROLE_MASTER）；uint8  Value=2  OutDataTypeStr=uint8
  C_ZeroU8 : Constant  Description=常量 0（LANE_STS_INITIALISING）；uint8  Value=0  OutDataTypeStr=uint8
  Logic_OrFail : Logic  Description=远程禁用或关闭 -> FAILED  Operator=OR  IconShape=distinctive  AllPortsSameDT=off  OutDataTypeStr=boolean
  Logic_OrInit : Logic  Description=远程 UNKNOWN/INIT -> INITIALISING  Operator=OR  IconShape=distinctive  AllPortsSameDT=off  OutDataTypeStr=boolean
  Relop_ActvMaster : RelationalOperator  Description=活动控制器：本链路角色==MASTER  Operator===  OutDataTypeStr=boolean  RndMeth=Simplest  InputSameDT=off
  Relop_RmtDisabled : RelationalOperator  Description=远程角色==DISABLED  Operator===  OutDataTypeStr=boolean  RndMeth=Simplest  InputSameDT=off
  Relop_RmtFitnessInvalid : RelationalOperator  Description=远程健康度==255（无效）-> HB_LOST  Operator===  OutDataTypeStr=boolean  RndMeth=Simplest  InputSameDT=off
  Relop_RmtInit : RelationalOperator  Description=远程角色==INIT  Operator===  OutDataTypeStr=boolean  RndMeth=Simplest  InputSameDT=off
  Relop_RmtShutdown : RelationalOperator  Description=远程角色==SHUTTING_DOWN  Operator===  OutDataTypeStr=boolean  RndMeth=Simplest  InputSameDT=off
  Relop_RmtUnknown : RelationalOperator  Description=远程角色==UNKNOWN  Operator===  OutDataTypeStr=boolean  RndMeth=Simplest  InputSameDT=off
  Switch_StsFail : Switch  Description=状态映射优先级 1：禁用/关闭 -> FAILED(3)  Criteria=u2 > Threshold  SaturateOnIntegerOverflow=off  InputSameDT=off
  Switch_StsHbLost : Switch  Description=状态映射优先级 2：健康度无效 -> HB_LOST(2)  Criteria=u2 > Threshold  SaturateOnIntegerOverflow=off  InputSameDT=off
  Switch_StsInit : Switch  Description=状态映射优先级 3：UNKNOWN/INIT -> INITIALISING(0)，否则 OPERATING(1)  Criteria=u2 > Threshold  SaturateOnIntegerOverflow=off  InputSameDT=off
  bActvCtrlr : Outport  Description=活动控制器实例标志（角色==MASTER）；类型 boolean
  u8RmtLaneSts : Outport  Description=远控制链路状态；类型 uint8；范围 0..3  Port=2
  bLaneSwtgInProgs : Outport  Description=控制链路切换进行中标志（直通）；类型 boolean  Port=3
  u8LaneRole : Outport  Description=本控制链路角色（直通）；类型 uint8；范围 0..6  Port=4
  wires:
  u8LaneRoleIn/1 -> u8LaneRole/1, Relop_ActvMaster/1
  C_TwoU8/1 -> Relop_ActvMaster/2, Switch_StsHbLost/1
  Relop_ActvMaster/1 -> bActvCtrlr/1
  u8RmtLaneRole/1 -> Relop_RmtInit/1, Relop_RmtUnknown/1, Relop_RmtShutdown/1, Relop_RmtDisabled/1
  C_FiveU8/1 -> Relop_RmtDisabled/2
  C_SixU8/1 -> Relop_RmtShutdown/2
  Relop_RmtDisabled/1 -> Logic_OrFail/1
  Relop_RmtShutdown/1 -> Logic_OrFail/2
  C_ThreeU8/1 -> Switch_StsFail/1
  Logic_OrFail/1 -> Switch_StsFail/2
  Switch_StsHbLost/1 -> Switch_StsFail/3
  u8RmtFitnessScore/1 -> Relop_RmtFitnessInvalid/1
  C_Max255U8/1 -> Relop_RmtFitnessInvalid/2
  Relop_RmtFitnessInvalid/1 -> Switch_StsHbLost/2
  Switch_StsInit/1 -> Switch_StsHbLost/3
  C_ZeroU8/1 -> Relop_RmtUnknown/2, Switch_StsInit/1
  C_OneU8/1 -> Relop_RmtInit/2, Switch_StsInit/3
  Relop_RmtUnknown/1 -> Logic_OrInit/1
  Relop_RmtInit/1 -> Logic_OrInit/2
  Logic_OrInit/1 -> Switch_StsInit/2
  Switch_StsFail/1 -> u8RmtLaneSts/1
  bLaneSwtgInProgsIn/1 -> bLaneSwtgInProgs/1

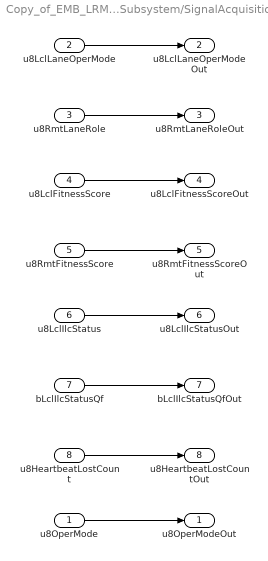
== system Copy_of_EMB_LRM_LaneRoleManager/MainSubsystem/SignalAcquisition ==
  u8OperMode : Inport  Description=系统运行模式（直通）；类型 uint8；单位 -；范围 0..5  OutDataTypeStr=uint8
  u8LclLaneOperMode : Inport  Description=本控制链路运行模式（直通）；类型 uint8；单位 -；范围 0..5  Port=2  OutDataTypeStr=uint8
  u8RmtLaneRole : Inport  Description=远控制链路当前角色（直通）；类型 uint8；单位 -；范围 0..6  Port=3  OutDataTypeStr=uint8
  u8LclFitnessScore : Inport  Description=本控制链路健康度得分（直通）；类型 uint8；单位 -；范围 0..255  Port=4  OutDataTypeStr=uint8
  u8RmtFitnessScore : Inport  Description=远控制链路健康度得分（直通）；类型 uint8；单位 -；范围 0..255  Port=5  OutDataTypeStr=uint8
  u8LclIlcStatus : Inport  Description=本控制链路 ILC 状态（直通）；类型 uint8；单位 -；范围 0..2  Port=6  OutDataTypeStr=uint8
  bLclIlcStatusQf : Inport  Description=本控制链路 ILC 状态信号质量（直通）；类型 boolean；单位 -；范围 0..1  Port=7  OutDataTypeStr=boolean
  u8HeartbeatLostCount : Inport  Description=心跳丢失计数（直通）；类型 uint8；单位 -；范围 0..255  Port=8  OutDataTypeStr=uint8
  u8OperModeOut : Outport  Description=系统运行模式（直通输出）；类型 uint8；单位 -；范围 0..5
  u8LclLaneOperModeOut : Outport  Description=本控制链路运行模式（直通输出）；类型 uint8；单位 -；范围 0..5  Port=2
  u8RmtLaneRoleOut : Outport  Description=远控制链路当前角色（直通输出）；类型 uint8；单位 -；范围 0..6  Port=3
  u8LclFitnessScoreOut : Outport  Description=本控制链路健康度得分（直通输出）；类型 uint8；单位 -；范围 0..255  Port=4
  u8RmtFitnessScoreOut : Outport  Description=远控制链路健康度得分（直通输出）；类型 uint8；单位 -；范围 0..255  Port=5
  u8LclIlcStatusOut : Outport  Description=本控制链路 ILC 状态（直通输出）；类型 uint8；单位 -；范围 0..2  Port=6
  bLclIlcStatusQfOut : Outport  Description=本控制链路 ILC 状态信号质量（直通输出）；类型 boolean；单位 -；范围 0..1  Port=7
  u8HeartbeatLostCountOut : Outport  Description=心跳丢失计数（直通输出）；类型 uint8；单位 -；范围 0..255  Port=8
  wires:
  u8HeartbeatLostCount/1 -> u8HeartbeatLostCountOut/1
  bLclIlcStatusQf/1 -> bLclIlcStatusQfOut/1
  u8LclIlcStatus/1 -> u8LclIlcStatusOut/1
  u8RmtFitnessScore/1 -> u8RmtFitnessScoreOut/1
  u8LclFitnessScore/1 -> u8LclFitnessScoreOut/1
  u8RmtLaneRole/1 -> u8RmtLaneRoleOut/1
  u8LclLaneOperMode/1 -> u8LclLaneOperModeOut/1
  u8OperMode/1 -> u8OperModeOut/1

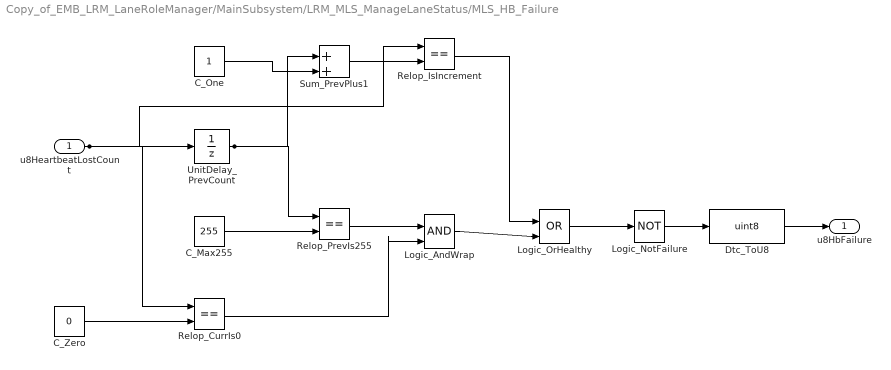
== system Copy_of_EMB_LRM_LaneRoleManager/MainSubsystem/LRM_MLS_ManageLaneStatus/MLS_HB_Failure ==
  u8HeartbeatLostCount : Inport  Description=心跳丢失计数；类型 uint8；范围 0..255  OutDataTypeStr=uint8
  C_Max255 : Constant  Description=最大值常量 255；uint8  Value=255  OutDataTypeStr=uint8
  C_One : Constant  Description=递增步长常量 1；uint8  OutDataTypeStr=uint8
  C_Zero : Constant  Description=零常量；uint8  Value=0  OutDataTypeStr=uint8
  Dtc_ToU8 : DataTypeConversion  Description=boolean 转 uint8 输出  OutDataTypeStr=uint8  SaturateOnIntegerOverflow=off  RndMeth=Floor
  Logic_AndWrap : Logic  Description=回卷检测：上一周期==255 且当前==0  IconShape=distinctive  AllPortsSameDT=off  OutDataTypeStr=boolean
  Logic_NotFailure : Logic  Description=故障条件：健康条件取反  Operator=NOT  Inputs=1  IconShape=distinctive  AllPortsSameDT=off  OutDataTypeStr=boolean
  Logic_OrHealthy : Logic  Description=健康条件：正常递增 或 回卷  Operator=OR  IconShape=distinctive  AllPortsSameDT=off  OutDataTypeStr=boolean
  Relop_CurrIs0 : RelationalOperator  Description=当前计数 == 0  Operator===  OutDataTypeStr=boolean  RndMeth=Simplest  InputSameDT=off
  Relop_IsIncrement : RelationalOperator  Description=当前计数 == 上一周期+1（正常递增）  Operator===  OutDataTypeStr=boolean  RndMeth=Simplest  InputSameDT=off
  Relop_PrevIs255 : RelationalOperator  Description=上一周期计数 == 255  Operator===  OutDataTypeStr=boolean  RndMeth=Simplest  InputSameDT=off
  Sum_PrevPlus1 : Sum  Description=上一周期计数 +1（uint8 溢出自动回卷）  Inputs=|++
  UnitDelay_PrevCount : UnitDelay  Description=保存上一周期心跳丢失计数，用于判定连续递增  SampleTime=-1  HasFrameUpgradeWarning=on
  u8HbFailure : Outport  Description=心跳丢失故障判断；类型 uint8；范围 0..1 (0=Not Failure,1=Failure)
  wires:
  Dtc_ToU8/1 -> u8HbFailure/1
  Logic_NotFailure/1 -> Dtc_ToU8/1
  Logic_OrHealthy/1 -> Logic_NotFailure/1
  Logic_AndWrap/1 -> Logic_OrHealthy/2
  Relop_IsIncrement/1 -> Logic_OrHealthy/1
  Relop_CurrIs0/1 -> Logic_AndWrap/2
  Relop_PrevIs255/1 -> Logic_AndWrap/1
  C_Zero/1 -> Relop_CurrIs0/2
  C_Max255/1 -> Relop_PrevIs255/2
  Sum_PrevPlus1/1 -> Relop_IsIncrement/2
  C_One/1 -> Sum_PrevPlus1/2
  UnitDelay_PrevCount/1 -> Sum_PrevPlus1/1, Relop_PrevIs255/1
  u8HeartbeatLostCount/1 -> UnitDelay_PrevCount/1, Relop_IsIncrement/1, Relop_CurrIs0/1
